simulink model "Model"  (R2015b)
settings: Solver=VariableStepAuto  StartTime=0.0  StopTime=20  RelTol=1e-3
libraries: sh_lib x9, nesl_utility x5, fl_lib x3
settings Model: Creator=s3blanch  LastModifiedBy=s3blanch
settings HardwareCC: TargetBitPerPointer=64  TargetLongLongMode=on  TargetIntDivRoundTo=Zero  TargetEndianess=LittleEndian  TargetWordSize=64  TargetHWDeviceType=MATLAB Host  ProdEqTarget=off
settings RTWCC: TargetLang=C++
settings GRTTargetCC: MultiInstanceERTCode=on  CodeInterfacePackaging=C++ class
settings SimscapeCC: SimscapeLogType=all

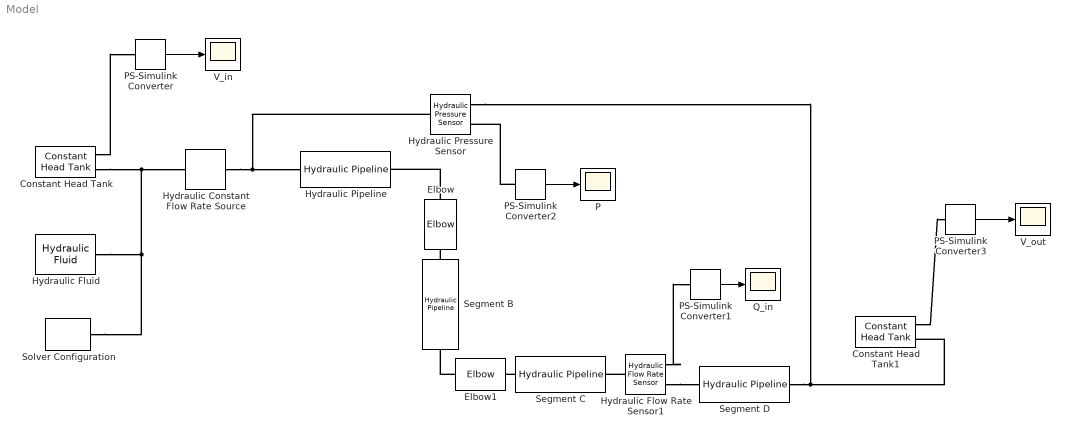
== system Model ==
  Constant Head Tank : sh_lib/Low-Pressure Blocks/Constant Head Tank  press=0 Pa  fluid_level=0 m  init_volume=V gal  pipe_diam=ID in  loss_coeff=1.2  gravity_accel=9.80665 m/s^2  pipe_area=0 m^2  C_d=0  p_cr=1 Pa
  Constant Head Tank1 : sh_lib/Low-Pressure Blocks/Constant Head Tank  press=0 Pa  fluid_level=0 m  init_volume=0 m^3  pipe_diam=ID in  loss_coeff=1.2  gravity_accel=9.80665 m/s^2  pipe_area=0 m^2  C_d=0  p_cr=1 Pa
  Elbow : sh_lib/Local Hydraulic Resistances/Elbow  elbow_diam=ID in  elbow_angle=90 deg  elbow_type=1  Re_cr=80
  Elbow1 : sh_lib/Local Hydraulic Resistances/Elbow  elbow_diam=ID in  elbow_angle=90 deg  elbow_type=1  Re_cr=80
  Hydraulic Constant Flow Rate Source : fl_lib/Hydraulic/Hydraulic Sources/Hydraulic Constant Flow Rate Source  commanded_flow_rate=Q gpm
  Hydraulic Flow Rate Sensor1 : fl_lib/Hydraulic/Hydraulic Sensors/Hydraulic Flow Rate Sensor
  Hydraulic Fluid : sh_lib/Hydraulic Utilities/Hydraulic Fluid  DataSource=1  SelFluid=11  SysTemp=25 c  TrapAir=0.005  ViscDerFactor=1  range_error=2
  Hydraulic Pipeline : sh_lib/Pipelines/Hydraulic Pipeline  cs_type=1  d_in=ID in  area=1e-4 m^2  D_h=0.0112 m  s_factor=S  length=La ft  length_ad=0 m  roughness=esp m  Re_lam=2e+3  Re_turb=4e+3  wall_type=1  pr_r_coef=2e-12 m/Pa  time_const=0.01 s  k_sh=1.4  initial_pressure=0 Pa
  Hydraulic Pressure Sensor : fl_lib/Hydraulic/Hydraulic Sensors/Hydraulic Pressure Sensor
  P : Scope
  PS-Simulink Converter : nesl_utility/PS-Simulink Converter  PhysicalDomain=network_engine_domain  SubClassName=ps_output  LeftPortType=input  RightPortType=output  PseudoPeriodic=off  Frequencies=[]  Unit=gal  AffineConversion=off
  PS-Simulink Converter1 : nesl_utility/PS-Simulink Converter  PhysicalDomain=network_engine_domain  SubClassName=ps_output  LeftPortType=input  RightPortType=output  PseudoPeriodic=off  Frequencies=[]  Unit=gpm  AffineConversion=off
  PS-Simulink Converter2 : nesl_utility/PS-Simulink Converter  PhysicalDomain=network_engine_domain  SubClassName=ps_output  LeftPortType=input  RightPortType=output  PseudoPeriodic=off  Frequencies=[]  Unit=psi  AffineConversion=off
  PS-Simulink Converter3 : nesl_utility/PS-Simulink Converter  PhysicalDomain=network_engine_domain  SubClassName=ps_output  LeftPortType=input  RightPortType=output  PseudoPeriodic=off  Frequencies=[]  Unit=1  AffineConversion=off
  Q_in : Scope
  Segment B : sh_lib/Pipelines/Hydraulic Pipeline  cs_type=1  d_in=ID in  area=1e-4 m^2  D_h=0.0112 m  s_factor=S  length=Lb ft  length_ad=0 m  roughness=esp m  Re_lam=2e+3  Re_turb=4e+3  wall_type=1  pr_r_coef=2e-12 m/Pa  time_const=0.01 s  k_sh=1.4  initial_pressure=0 Pa
  Segment C : sh_lib/Pipelines/Hydraulic Pipeline  cs_type=1  d_in=ID in  area=1e-4 m^2  D_h=0.0112 m  s_factor=S  length=Lc ft  length_ad=Leq ft  roughness=esp m  Re_lam=2e+3  Re_turb=4e+3  wall_type=1  pr_r_coef=2e-12 m/Pa  time_const=0.01 s  k_sh=1.4  initial_pressure=0 Pa
  Segment D : sh_lib/Pipelines/Hydraulic Pipeline  cs_type=1  d_in=ID in  area=1e-4 m^2  D_h=0.0112 m  s_factor=S  length=Ld ft  length_ad=0 m  roughness=esp m  Re_lam=2e+3  Re_turb=4e+3  wall_type=1  pr_r_coef=2e-12 m/Pa  time_const=0.01 s  k_sh=1.4  initial_pressure=0 Pa
  Solver Configuration : nesl_utility/Solver Configuration  PhysicalDomain=network_engine_domain  SubClassName=solver  LeftPortType=input  RightPortType=generic  Accelerate=off  Tones=[]  Harmonics=[]  SimulateNoise=off  Profile=off  UseLocalSampling=off  EnableSwitchedLinearOptims=on  FrequencyDomain=off  UseCCode=off  RelTol=0.001  AbsTol=1e-06  MinStep=1e-09  ToWorkspace=off  RevertToSquareIcSolve=off  NumHomotopyIterations=100  PhasorMode=off  PhasorModeNumHarmonics=1  DoDC=off  ResidualTolerance=1e-9  UseLocalSolver=off  LocalSolverChoice=NE_BACKWARD_EULER_ADVANCER  LocalSolverSampleTime=0.001  DoFixedCost=off  MaxNonlinIter=3  MaxModeIter=2  LinearAlgebra=Sparse  DelaysMemoryBudget=1024  AutomaticFiltering=on  FilteringTimeConstant=0.001
  V_in : Scope
  V_out : Scope
  wires:
  PS-Simulink Converter/1 -> V_in/1
  PS-Simulink Converter1/1 -> Q_in/1
  PS-Simulink Converter2/1 -> P/1
  PS-Simulink Converter3/1 -> V_out/1
  connections:
  Elbow/LConn1 -- Hydraulic Pipeline/RConn1
  Elbow1/LConn1 -- Segment B/RConn1
  Segment B/LConn1 -- Elbow/RConn1
  Segment C/LConn1 -- Elbow1/RConn1
  Hydraulic Fluid/RConn1 -- Solver Configuration/RConn1 -- Constant Head Tank/RConn2 -- Hydraulic Constant Flow Rate Source/RConn1
  Constant Head Tank/RConn1 -- PS-Simulink Converter/LConn1
  Hydraulic Flow Rate Sensor1/RConn1 -- PS-Simulink Converter1/LConn1
  PS-Simulink Converter2/LConn1 -- Hydraulic Pressure Sensor/RConn2
  Constant Head Tank1/RConn1 -- PS-Simulink Converter3/LConn1
  Hydraulic Constant Flow Rate Source/LConn1 -- Hydraulic Pressure Sensor/LConn1 -- Hydraulic Pipeline/LConn1
  Hydraulic Flow Rate Sensor1/LConn1 -- Segment C/RConn1
  Constant Head Tank1/RConn2 -- Segment D/RConn1 -- Hydraulic Pressure Sensor/RConn1
  Hydraulic Flow Rate Sensor1/RConn2 -- Segment D/LConn1
